simulink library "UR3_Lib"  (R2017a)
settings: Solver=VariableStepAuto  StartTime=0.0  StopTime=10.0  RelTol=1e-3
settings Model: Creator=dscat  LastModifiedBy=dscat

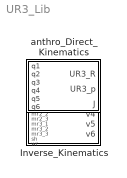
== system UR3_Lib ==
  Inverse_Kinematics : MATLAB Function  TreatAsAtomicUnit=on
  anthro_Direct_Kinematics : MATLAB Function  TreatAsAtomicUnit=on

== matlab function UR3_Lib/Inverse_Kinematics ==
  data: el input; v1 output; mp1 input; mp2 input; mp3 input; mr1_1 input; mr1_2 input; mr1_3 input; mr2_1 input; mr2_2 input; mr2_3 input; mr3_1 input; mr3_2 input; mr3_3 input; sh input; wr input; v2 output; v3 output; v4 output; v5 output; v6 output
function [v1,v2,v3,v4,v5,v6] = Inverse_Kinematics(el,mp1,mp2,mp3,mr1_1,mr1_2,mr1_3,mr2_1,mr2_2,mr2_3,mr3_1,mr3_2,mr3_3,sh,wr)
%#codegen

%    This function was generated by the Symbolic Math Toolbox version 7.2.
%    24-Apr-2018 21:19:32

t6 = mr1_3.*(4.1e1./5.0e2);
t2 = mp1-t6;
t9 = mr2_3.*(4.1e1./5.0e2);
t3 = mp2-t9;
t4 = pi.*(1.0./2.0);
t5 = mp2.*1i;
t7 = mr2_3.*-8.2e-2i;
t8 = t2.^2;
t10 = t3.^2;
t11 = t8+t10;
t12 = 1.0./sqrt(t11);
t13 = t12.*(1.1e1./1.0e2);
t14 = acos(t13);
t15 = sh.*t14;
v1 = t4+t15+angle(mp1-mr1_3.*(4.1e1./5.0e2)+t5+t7);
if nargout > 1
    t16 = mp1+t5-t6+t7;
    t17 = angle(t16);
    t18 = t4+t15+t17;
    t19 = cos(t18);
    t20 = sin(t18);
    t21 = t19.^2;
    t22 = t20.^2;
    t23 = t21+t22;
    t24 = 1.0./t23;
    t25 = mp1.*t20.*(5.0e2./4.1e1);
    t31 = mp2.*t19.*(5.0e2./4.1e1);
    t26 = t25-t31-5.5e1./4.1e1;
    t27 = acos(t26);
    t28 = t27.*wr;
    t29 = sin(t28);
    t30 = 1.0./t29;
    t32 = cos(t28);
    t33 = mr1_2.*t20;
    t38 = mr2_2.*t19;
    t34 = t33-t38;
    t35 = mr1_1.*t20;
    t37 = mr2_1.*t19;
    t36 = t35-t37;
    t44 = t30.*t34;
    t39 = real(-t44);
    t42 = t30.*t36;
    t40 = imag(-t42);
    t41 = t39-t40;
    t116 = t30.*(t33-t38).*-1i;
    t43 = -t116;
    t45 = -t42+t43;
    t46 = abs(t45);
    t47 = t32.^2;
    t48 = real(-t42);
    t49 = imag(-t44);
    t50 = t48+t49;
    t51 = 1.0./t46.^2;
    t52 = t29.^2;
    t53 = t50.^2;
    t54 = t41.^2;
    t55 = 1.0./t46;
    t56 = t47.*t51.*t53;
    t57 = t51.*t52.*t53;
    t58 = t47.*t51.*t54;
    t59 = t51.*t52.*t54;
    t60 = t56+t57+t58+t59;
    t61 = 1.0./t60;
    t63 = t47.*t50.*t55.*8.3e1;
    t64 = t29.*t41.*t55.*1.1e2;
    t65 = t50.*t52.*t55.*8.3e1;
    t66 = t63-t64+t65;
    t67 = t29.*t50.*t55.*1.1e2;
    t68 = t47+t52;
    t69 = 1.0./t68;
    t70 = t32.*5.5e1;
    t71 = t47.*4.1e1;
    t72 = t52.*4.1e1;
    t73 = t70+t71+t72;
    t81 = mr1_1.*t19.*t24;
    t82 = mr2_1.*t20.*t24;
    t83 = t81+t82;
    t84 = mp1.*t19.*t24;
    t85 = mp2.*t20.*t24;
    t86 = mr1_3.*t19.*t24;
    t87 = mr2_3.*t20.*t24;
    t88 = t86+t87;
    t89 = t69.*t73.*t88.*(1.0./5.0e2);
    t90 = mr1_2.*t19.*t24;
    t91 = mr2_2.*t20.*t24;
    t92 = t90+t91;
    t93 = t61.*t66.*t92.*(1.0./1.0e3);
    t62 = t84+t85-t89-t93+t61.*t83.*(t67+(t41.*t52.*8.3e1)./abs(t43-t30.*t36)+(t41.*t47.*8.3e1)./abs(t30.*t34.*1i-t30.*t36)).*(1.0./1.0e3);
    t75 = mr3_2.*t61.*t66.*(1.0./1.0e3);
    t76 = t41.*t47.*t55.*8.3e1;
    t77 = t41.*t52.*t55.*8.3e1;
    t78 = t67+t76+t77;
    t79 = mr3_1.*t61.*t78.*(1.0./1.0e3);
    t80 = mr3_3.*t69.*t73.*(1.0./5.0e2);
    t74 = mp3-t75+t79-t80;
    t97 = t61.*t78.*t83.*(1.0./1.0e3);
    t94 = t84+t85-t89-t93+t97;
    t95 = t74.^2;
    t98 = t94.^2;
    t100 = t98.*9.620564919572077;
    t101 = t95.*9.620564919572077;
    t96 = t100+t101-1.009245362887709;
    t99 = t95.*(1.25e2./6.1e1);
    t102 = t96.^2;
    t103 = -t102+1.0;
    t104 = sqrt(t103);
    t105 = t95+t98;
    t106 = 1.0./t105;
    t107 = el.*t104.*1i;
    t108 = t100+t101+t107-1.009245362887709;
    t109 = angle(t108);
    t110 = t98.*(1.25e2./6.1e1);
    t111 = t99+t110+2.903073770491803e-2;
    t112 = t94.*t111;
    t113 = el.*t74.*t104.*(2.13e2./1.0e3);
    t114 = t112+t113;
    t115 = t106.*t114.*1i;
    v2 = -angle(t115+t106.*(t74.*(t99+t62.^2.*(1.25e2./6.1e1)+2.903073770491803e-2)-el.*t94.*t104.*(2.13e2./1.0e3)));
end
if nargout > 2
    v3 = t109;
end
if nargout > 3
    v4 = -t109+angle(t115+t106.*(t74.*t111-el.*t94.*t104.*(2.13e2./1.0e3)))+angle(-mr3_1.*t41.*t55+mr3_2.*t50.*t55+mr1_1.*t19.*t41.*t55.*1i-mr1_2.*t19.*t50.*t55.*1i+mr2_1.*t20.*t41.*t55.*1i-mr2_2.*t20.*t50.*t55.*1i);
end
if nargout > 4
    v5 = t28;
end
if nargout > 5
    v6 = angle(t116+t30.*(t35-t37));
end

== matlab function UR3_Lib/anthro_Direct_Kinematics ==
  data: q1 input; UR3_R output; q2 input; q3 input; q4 input; q5 input; q6 input; UR3_p output; J output
function [UR3_R,UR3_p,J] = anthro_Direct_Kinematics(q1,q2,q3,q4,q5,q6)
%#codegen

%    This function was generated by the Symbolic Math Toolbox version 7.2.
%    24-Apr-2018 21:14:01

t2 = cos(q1);
t3 = cos(q2);
t4 = cos(q5);
t5 = cos(q3);
t6 = sin(q4);
t7 = cos(q4);
t8 = sin(q2);
t9 = sin(q3);
t10 = sin(q6);
t11 = sin(q1);
t12 = sin(q5);
t13 = t11.*t12;
t14 = t2.*t3.*t4.*t6.*t9;
t15 = t2.*t4.*t5.*t6.*t8;
t16 = t2.*t4.*t7.*t8.*t9;
t17 = t13+t14+t15+t16-t2.*t3.*t4.*t5.*t7;
t18 = q2+q3+q4;
t19 = sin(t18);
t20 = cos(q6);
t21 = t3.*t4.*t6.*t9.*t11;
t22 = t4.*t5.*t6.*t8.*t11;
t23 = t4.*t7.*t8.*t9.*t11;
t24 = t21+t22+t23-t2.*t12-t3.*t4.*t5.*t7.*t11;
t25 = q2+q3+q4+q6;
t26 = q2+q3+q4-q6;
t27 = q2+q3+q4+q5;
t28 = cos(t27);
t29 = q2+q3+q4-q5;
t30 = cos(t29);
t31 = t6.*t8.*t9.*t11.*(8.3e1./1.0e3);
t32 = t3.*t5.*t7.*t11.*t12.*(4.1e1./5.0e2);
t33 = cos(t18);
t34 = t33.*(8.3e1./1.0e3);
t35 = q2+q3;
t36 = cos(t35);
t37 = t36.*(2.13e2./1.0e3);
t38 = t3.*(6.1e1./2.5e2);
t39 = t30.*(4.1e1./1.0e3);
t41 = t28.*(4.1e1./1.0e3);
t40 = t34+t37+t38+t39-t41;
t42 = t2.*t4.*(4.1e1./5.0e2);
t43 = t3.*t5.*t6.*t11.*(8.3e1./1.0e3);
t44 = t3.*t7.*t9.*t11.*(8.3e1./1.0e3);
t45 = t5.*t7.*t8.*t11.*(8.3e1./1.0e3);
t46 = t3.*t6.*t9.*t11.*t12.*(4.1e1./5.0e2);
t47 = t5.*t6.*t8.*t11.*t12.*(4.1e1./5.0e2);
t48 = t7.*t8.*t9.*t11.*t12.*(4.1e1./5.0e2);
t49 = t34+t39-t41;
t50 = t3.*t5.*t7.*t11.*t12;
t51 = t30.*(1.0./2.0);
t52 = t11.*(1.1e1./1.0e2);
t53 = t4.*t11.*(4.1e1./5.0e2);
t54 = t2.*t6.*t8.*t9.*(8.3e1./1.0e3);
t55 = t2.*t3.*t5.*t7.*t12.*(4.1e1./5.0e2);
t60 = t2.*t3.*t5.*t6.*(8.3e1./1.0e3);
t61 = t2.*t3.*t7.*t9.*(8.3e1./1.0e3);
t62 = t2.*t5.*t7.*t8.*(8.3e1./1.0e3);
t63 = t2.*t3.*t6.*t9.*t12.*(4.1e1./5.0e2);
t64 = t2.*t5.*t6.*t8.*t12.*(4.1e1./5.0e2);
t65 = t2.*t7.*t8.*t9.*t12.*(4.1e1./5.0e2);
t75 = t2.*t8.*(6.1e1./2.5e2);
t76 = t2.*t3.*t9.*(2.13e2./1.0e3);
t77 = t2.*t5.*t8.*(2.13e2./1.0e3);
t56 = t52+t53+t54+t55-t60-t61-t62-t63-t64-t65-t75-t76-t77;
t57 = t34+t37+t39-t41;
t58 = q1+q2+q3+q4;
t59 = -q1+q2+q3+q4;
t66 = t4.*t11;
t67 = t2.*t3.*t5.*t7.*t12;
UR3_R = reshape([t17.*t20+t2.*t10.*t19,t20.*t24+t10.*t11.*t19,sin(t25).*(-1.0./2.0)+sin(t26).*(1.0./2.0)-t4.*t19.*t20,-t10.*t17+t2.*t19.*t20,-t10.*t24+t11.*t19.*t20,cos(t25).*(-1.0./2.0)-cos(t26).*(1.0./2.0)+t4.*t10.*t19,t66+t67-t2.*t3.*t6.*t9.*t12-t2.*t5.*t6.*t8.*t12-t2.*t7.*t8.*t9.*t12,t50-t2.*t4-t3.*t6.*t9.*t11.*t12-t5.*t6.*t8.*t11.*t12-t7.*t8.*t9.*t11.*t12,t28.*(-1.0./2.0)+t51],[3,3]);
if nargout > 1
    UR3_p = [t56;t2.*(-1.1e1./1.0e2)+t31+t32-t2.*t4.*(4.1e1./5.0e2)-t8.*t11.*(6.1e1./2.5e2)-t3.*t9.*t11.*(2.13e2./1.0e3)-t5.*t8.*t11.*(2.13e2./1.0e3)-t3.*t5.*t6.*t11.*(8.3e1./1.0e3)-t3.*t7.*t9.*t11.*(8.3e1./1.0e3)-t5.*t7.*t8.*t11.*(8.3e1./1.0e3)-t3.*t6.*t9.*t11.*t12.*(4.1e1./5.0e2)-t5.*t6.*t8.*t11.*t12.*(4.1e1./5.0e2)-t7.*t8.*t9.*t11.*t12.*(4.1e1./5.0e2);t40];
end
if nargout > 2
    t68 = t28.*(1.0./2.0);
    t69 = t51-t68;
    t70 = t2.*(1.1e1./1.0e2);
    t71 = t8.*t11.*(6.1e1./2.5e2);
    t72 = t3.*t9.*t11.*(2.13e2./1.0e3);
    t73 = t5.*t8.*t11.*(2.13e2./1.0e3);
    t74 = -t31-t32+t42+t43+t44+t45+t46+t47+t48+t70+t71+t72+t73;
    t78 = sin(t35);
    t79 = t78.*2.13e2;
    t80 = t8.*2.44e2;
    t81 = t79+t80;
    t82 = cos(t58);
    t83 = t82.*(1.0./2.0);
    t84 = cos(t59);
    t104 = t84.*(1.0./2.0);
    t85 = t83-t104;
    t86 = -t53-t54-t55+t60+t61+t62+t63+t64+t65;
    t87 = sin(t58);
    t88 = t87.*(1.0./2.0);
    t89 = sin(t59);
    t90 = t89.*(1.0./2.0);
    t91 = t88+t90;
    t92 = -t31-t32+t42+t43+t44+t45+t46+t47+t48;
    t93 = -t53-t55+t63+t64+t65;
    t94 = t2.*t4;
    t95 = t3.*t6.*t9.*t11.*t12;
    t96 = t5.*t6.*t8.*t11.*t12;
    t97 = t7.*t8.*t9.*t11.*t12;
    t98 = -t50+t94+t95+t96+t97;
    t99 = t2.*t3.*t6.*t9.*t12;
    t100 = t2.*t5.*t6.*t8.*t12;
    t101 = t2.*t7.*t8.*t9.*t12;
    t102 = -t66-t67+t99+t100+t101;
    t103 = -t32+t42+t46+t47+t48;
    J = reshape([t74,t56,0.0,0.0,0.0,1.0,-t2.*t40,-t11.*t40,-t11.*t74-t2.*(-t52-t53-t54-t55+t60+t61+t62+t63+t64+t65+t75+t76+t77),t11,-t2,0.0,-t2.*t57,-t11.*t57,-t2.*(-t52-t53-t54-t55+t60+t61+t62+t63+t64+t65+t76+t77)-t11.*(-t31-t32+t42+t43+t44+t45+t46+t47+t48+t70+t72+t73),t11,-t2,0.0,-t2.*t49,-t11.*t49,-t11.*(-t31-t32+t42+t43+t44+t45+t46+t47+t48+t70+t71+t72+t73-t11.*t81.*(1.0./1.0e3))-t2.*(-t52-t53-t54-t55+t60+t61+t62+t63+t64+t65+t75+t76+t77-t2.*t81.*(1.0./1.0e3)),t11,-t2,0.0,t33.*t92+t49.*t85,-t33.*t86+t49.*t91,t85.*t86+t91.*t92,-t88-t90,t85,t33,t69.*t103-t98.*(t39-t41),-t69.*t93+t102.*(t39-t41),-t93.*t98+t102.*t103,t66+t67-t99-t100-t101,t50-t94-t95-t96-t97,t69],[6,6]);
end
